simulink model "acquisition"  (R2019a)
settings: Solver=ode1  StartTime=0.0  StopTime=Tf  FixedStep=Ts  RelTol=1e-3  EnableMultiTasking=on
values from neighbouring files (symbols this model uses):
  encoder_fw_resolution = 3    [acquisition_routine_generic_device.m]
  gear_ratio = 35/3    (= 11.6666666667)    [acquisition_routine_generic_device.m]
libraries: qbmove_library x2, dspsigops x2, qbmove_library_2017a x1, QB_pacer_lib x1
settings Model: Creator=Matteo  LastModifiedBy=Mattia
settings DataIOCC: LimitDataPoints=on  SaveFormat=Array  ReturnWorkspaceOutputs=off
settings OptimizationCC: LifeSpan=inf
settings DebuggingCC: UnderspecifiedInitializationDetection=Classic  MergeDetectMultiDrivingBlocksExec=none  SolverPrmCheckMsg=warning  StateNameClashWarn=warning  SFUnexpectedBacktrackingDiag=warning  SFNoUnconditionalDefaultTransitionDiag=warning  SFExecutionAtInitializationDiag=none  ArithmeticOperatorsInVariantConditions=warning
settings HardwareCC: ProdBitPerPointer=32  ProdBitPerSizeT=32  ProdBitPerPtrDiffT=32  ProdLargestAtomicFloat=None  ProdIntDivRoundTo=Undefined  ProdEndianess=Unspecified  ProdWordSize=32  ProdHWDeviceType=32-bit Generic
settings ModelReferenceCC: PropagateSignalLabelsOutOfModel=off
settings SFSimCC: SimUseLocalCustomCode=off
settings RTWCC: RTWUseLocalCustomCode=off
settings CodeAppCC: StateflowObjectComments=on
settings GRTTargetCC: TargetLangStandard=C89/C90 (ANSI)  GeneratePreprocessorConditionals=Disable all
settings ConfigComp: CovMetricSettings=dw  CovHtmlReporting=on  CovSaveCumulativeToWorkspaceVar=on  CovSaveSingleToWorkspaceVar=on  CovExternalEMLEnable=off

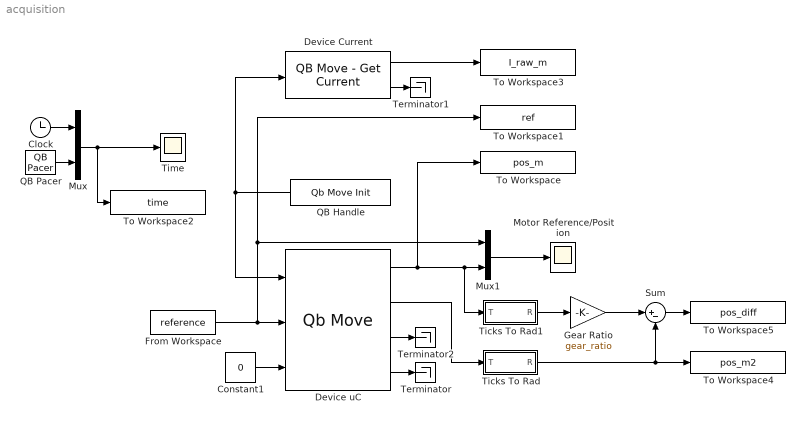
== system acquisition ==
  Clock : Clock
  Constant1 : Constant  Value=0
  Device Current : qbmove_library/QB Move - Get Current  ID=device_ID  CONTROL_MODE=Prime Movers Positions  DAISY_CHAINING=off
      settings: SourceProductName=Qb Move Library
  Device uC : qbmove_library_2017a/Qb Move  ID=device_ID  ACTIVE_COMM_DIRECTIONS=Both  CONTROL_MODE=Prime Movers Positions  DAISY_CHAINING=off  MAX_ANG=0  SW_LIMIT=inf  OFFSET=0  ACTIVATE=on  WDT=0.0  UNIT=TICK
  From Workspace : FromWorkspace  VariableName=reference  OutputAfterFinalValue=Holding final value
  Gear Ratio : Gain  Gain=gear_ratio
  Motor Reference/Position : Scope
  Mux : Mux  Inputs=2
  Mux1 : Mux  Inputs=2
  QB Handle : qbmove_library/Qb Move Init  NUMBER_OF_COM=COM_port  BAUD_RATE_COM=2000000
      settings: SourceProductName=Qb Move Library
  QB Pacer : QB_pacer_lib/QB Pacer  simTimePerRealTime=1
  Sum : Sum  Inputs=|+-
  Terminator : Terminator
  Terminator1 : Terminator
  Terminator2 : Terminator
  Ticks To Rad : Subsystem
  Ticks To Rad1 : Subsystem
  Time : Scope
  To Workspace : ToWorkspace  VariableName=pos_m  SaveFormat=Timeseries  SampleTime=-1
  To Workspace1 : ToWorkspace  VariableName=ref  SampleTime=-1
  To Workspace2 : ToWorkspace  VariableName=time  SampleTime=-1
  To Workspace3 : ToWorkspace  VariableName=I_raw_m  SaveFormat=Timeseries  SampleTime=-1
  To Workspace4 : ToWorkspace  VariableName=pos_m2  SaveFormat=Timeseries  SampleTime=-1
  To Workspace5 : ToWorkspace  VariableName=pos_diff  SaveFormat=Timeseries  SampleTime=-1
  wires:
  QB Handle/1 -> Device uC/1, Device Current/1
  QB Pacer/1 -> Mux/2
  Clock/1 -> Mux/1
  Mux/1 -> To Workspace2/1, Time/1
  Device uC/4 -> Terminator/1
  Device Current/2 -> Terminator1/1
  Device uC/3 -> Terminator2/1
  From Workspace/1 -> To Workspace1/1, Mux1/1, Device uC/2
  Device Current/1 -> To Workspace3/1
  Mux1/1 -> Motor Reference/Position/1
  Constant1/1 -> Device uC/3
  Sum/1 -> To Workspace5/1
  Device uC/1 -> Ticks To Rad1/1(T), Mux1/2, To Workspace/1
  Ticks To Rad/1(R) -> Sum/2, To Workspace4/1
  Device uC/2 -> Ticks To Rad/1(T)
  Ticks To Rad1/1(R) -> Gear Ratio/1
  Gear Ratio/1 -> Sum/1

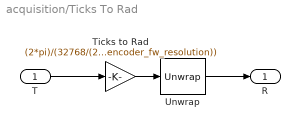
== system acquisition/Ticks To Rad ==
  T : Inport
  Ticks to Rad : Gain  Gain=(2*pi)/(32768/(2^encoder_fw_resolution))
  Unwrap : dspsigops/Unwrap  tol=pi  InputProcessing=Columns as channels (frame based)  running=off
  R : Outport
  wires:
  T/1 -> Ticks to Rad/1
  Ticks to Rad/1 -> Unwrap/1
  Unwrap/1 -> R/1

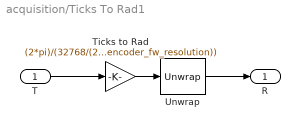
== system acquisition/Ticks To Rad1 ==
  T : Inport
  Ticks to Rad : Gain  Gain=(2*pi)/(32768/(2^encoder_fw_resolution))
  Unwrap : dspsigops/Unwrap  tol=pi  InputProcessing=Columns as channels (frame based)  running=off
  R : Outport
  wires:
  Unwrap/1 -> R/1
  Ticks to Rad/1 -> Unwrap/1
  T/1 -> Ticks to Rad/1
